simulink model "SIMULINK_FT_SRL_NZS_Tracking_R18b"  (R2018b)
settings: Solver=FixedStepAuto  StartTime=0.0  StopTime=sim_end_time  FixedStep=fixed_step_size  RelTol=1e-3
InitFcn:
  | start_uav_car_10
values from neighbouring files (symbols this model uses):
  a = 1    [start_uav_car_10.m]
  act_end = 2*pi/w1    (= 62.8318530718)    [start_uav_car_10.m]
  b = 1.8    [start_uav_car_10.m]
  battery_threshold = 20    [start_uav_car_10.m]
  bb = 1.2    [start_uav_car_10.m]
  delta_ = [delta_his(2:end,:); delta]    [adp_tracking.m]    (also in start_uav_car_10.m = zeros(N,1))
  draw_gif = false    [start_uav_car_10.m]
  fixed_step_size = 1/30    (= 0.0333333333333)    [start_uav_car_10.m]
  k = 0.2    [start_uav_car_10.m]
  KD_x = 0.000002    (= 2e-06)    [start_uav_car_10.m]
  KD_y = 0.00002    (= 2e-05)    [start_uav_car_10.m]
  kd_z = 0.02    [start_uav_car_10.m]
  KDD_x = 0.0008    [start_uav_car_10.m]
  KDD_y = 0.0008    [start_uav_car_10.m]
  KI_x = 0.000002    (= 2e-06)    [start_uav_car_10.m]
  KI_y = 0.000002    (= 2e-06)    [start_uav_car_10.m]
  ki_z = 0.002    [start_uav_car_10.m]
  KII_x = 0.000000    (= 0)    [start_uav_car_10.m]
  KII_y = 0.000    (= 0)    [start_uav_car_10.m]
  KP_x = 1.5    [start_uav_car_10.m]
  KP_y = 1.5    [start_uav_car_10.m]
  kp_z = 0.7    [start_uav_car_10.m]
  KPP_x = 0.4    [start_uav_car_10.m]
  KPP_y = 0.4    [start_uav_car_10.m]
  lmt = 0.5    [start_uav_car_10.m]
  omega = omega_(i,:)    [adp_tracking.m]    (also in start_uav_car_10.m = 0.3)
  omega_ = [omega_his(2:end,:); omega']    [adp_tracking.m]    (also in start_uav_car_10.m = zeros(N,l))
  R = 200*eye(2)    [adp_tracking.m]    (also in start_uav_car_10.m = 0.7)
  sim_end_time = 300    [start_uav_car_10.m]    (also in trjcar.m = 600)
  UAV_NUM = 1    [start_uav_car_10.m]
  Vel_Switch_1 = 1    [start_uav_car_10.m]
  Vel_Switch_10 = 1    [start_uav_car_10.m]
  Vel_Switch_11 = 1    [start_uav_car_10.m]
  Vel_Switch_12 = 1    [start_uav_car_10.m]
  Vel_Switch_13 = 1    [start_uav_car_10.m]
  Vel_Switch_14 = 1    [start_uav_car_10.m]
  Vel_Switch_15 = 1    [start_uav_car_10.m]
  Vel_Switch_16 = 1    [start_uav_car_10.m]
  Vel_Switch_17 = 1    [start_uav_car_10.m]
  Vel_Switch_18 = 1    [start_uav_car_10.m]
  Vel_Switch_19 = 1    [start_uav_car_10.m]
  Vel_Switch_2 = 1    [start_uav_car_10.m]
  Vel_Switch_20 = 1    [start_uav_car_10.m]
  Vel_Switch_3 = 1    [start_uav_car_10.m]
  Vel_Switch_4 = 1    [start_uav_car_10.m]
  Vel_Switch_5 = 1    [start_uav_car_10.m]
  Vel_Switch_6 = 1    [start_uav_car_10.m]
  Vel_Switch_7 = 1    [start_uav_car_10.m]
  Vel_Switch_8 = 1    [start_uav_car_10.m]
  Vel_Switch_9 = 1    [start_uav_car_10.m]
  W0 = 10*ones(l,1)    [start_uav_car_10.m]
  w1 = 0.1    [start_uav_car_10.m]
  w2 = 30    [start_uav_car_10.m]
  XMAX = 2.8    [start_uav_car_10.m]
  XMIN = -2.8    [start_uav_car_10.m]
  YMAX = 2.2    [start_uav_car_10.m]
  YMIN = -2.2    [start_uav_car_10.m]
  ys = ys_learned - ys_learned(1,:)    [start_uav_car_10.m]
  ys_learned = [-20 -19.9842645881 -19.9722755737 -19.9635643089 -19.9577075469 -19.9543235714 -19.9530686431 -19.9536337356 -19.9557415391 -19.9591437091 -19.9636183405 -19.9689676484 ... (12618 elements, 6309x2)]    [DMP_ref.mat]
  z_d_for_land = 1    [start_uav_car_10.m]
  ZMAX = 2.0    (= 2)    [start_uav_car_10.m]
  ZMIN = 0.7    [start_uav_car_10.m]
undefined symbols (not defined in the file or in its folder): droneyeeUAV2_NUM, droneyeeUAV3_NUM, droneyeeUAV4_NUM, droneyeeUAV5_NUM, uav10num, uav1num, uav2num, uav3num, uav4num, uav5num, uav6num, uav7num, uav8num, uav9num
libraries: simulink x121, aerolibanimutils x1
(part 11 of 11)

== matlab function SIMULINK_FT_SRL_NZS_Tracking_R18b/CMD_car1/CMD6/MATLAB Function1 ==
  settings: updateMethod=DISCRETE
  data: x_d input; y_d input; z_d input; timestamp input; x input; y input; z input; battery_status input; sim_time_end input; x_d_ output; battery_threshold input; z_d_for_land input; y_d_ output; z_d_ output; UAV_NUM input
function [x_d_, y_d_, z_d_] = fcn(x_d, y_d, z_d, timestamp, x,y,z,battery_status, sim_time_end,battery_threshold, z_d_for_land, UAV_NUM)
persistent s_x s_y s_z ready_land
if isempty(s_x)
    s_x = x;
end
if isempty(s_y)
    s_y = y;
end
if isempty(s_z)
    s_z = z;
end
if isempty(ready_land)
    ready_land = false;
end
    
battery_low = false;
for i = 1:UAV_NUM
    if battery_status(i) < battery_threshold
        battery_low = true;
        break;
    end
end
if sim_time_end - timestamp < 1
    tello_stop = true;
else
    tello_stop = false;
end
if battery_low || tello_stop
    if ~ready_land
        ready_land = true;
    end
    z_d_ = z_d_for_land;
    x_d_ = s_x;
    y_d_ = s_y;
else
   ready_land = false;
   s_x = x;
   s_y = y;
   x_d_ = x_d;
   y_d_ = y_d;
   z_d_ = z_d;
end

== matlab function SIMULINK_FT_SRL_NZS_Tracking_R18b/control system_UAV/MATLAB Function ==
  data: u input; y output
function y = fcn(u)
plot(u(1),u(2),"*");
hold on;
y = u;

== matlab function SIMULINK_FT_SRL_NZS_Tracking_R18b/防碰撞2/MATLAB Function ==
  settings: updateMethod=DISCRETE
  data: u1 input; xd output; u2 input; yd output; zd output; u3 input; u4 input; u5 input; flag input
function [xd,yd,zd] = fcn(u1,u2,u3,u4,u5,flag)
persistent xdd ydd zdd xtt ytt ztt;
k=u4;
totnum =10;
safedist =u3;%安全距离的平方
bang=u5;
xdd=zeros(totnum,1);
ydd=zeros(totnum,1);
zdd=zeros(totnum,1);
xt=zeros(totnum,1);
yt=zeros(totnum,1);
zt=zeros(totnum,1);
vx=xt;
vy=yt;
vz=zt;
xd=xt;
yd=yt;
zd=zt;
for i =1:1:totnum
    xt(i)=u2(12*(i-1)+1);
    yt(i)=u2(12*(i-1)+2);
    zt(i)=u2(12*(i-1)+3);
    xd(i)=u1(6*(i-1)+1);
    yd(i)=u1(6*(i-1)+2);
    zd(i)=u1(6*(i-1)+3);
    vx(i)=u2(12*(i-1)+10);
    vy(i)=u2(12*(i-1)+11);
    vz(i)=u2(12*(i-1)+12);
end
if flag==1
if isempty(xt)
    xtt = xt;
    ytt = yt;
    ztt = zt;
end
for i =1:1:(totnum-1)
    if xt(i)==0&&yt(i)==0&&zt(i)==0
        break
    end
    for j=(i+1):1:totnum
        if xt(j)==0&&yt(j)==0&&zt(j)==0
        break
        end
        dist=((xt(i)-xt(j))^2+(yt(i)-yt(j))^2+(zt(i)-zt(j))^2);
        sqrt_dist=sqrt((xt(i)-xt(j))^2+(yt(i)-yt(j))^2);
    if (dist>0)&&(sqrt(dist)<=bang)
%         xd(i)=xt(i);
%         yd(i)=yt(i);
%         zd(i)=0; %zt(i);
%         xd(j)=xt(j);
%         yd(j)=yt(j);
%         zd(j)=zt(j);        
%         xd(i)=xd(i)+k*(xt(i)-xt(j))*(safedist-dist);
%         yd(i)=yd(i)+k*(yt(i)-yt(j))*(safedist-dist);
        xdd(i)=xdd(i)+k*(xt(i)-xt(j))*(safedist-dist);
        ydd(i)=ydd(i)+k*(yt(i)-yt(j))*(safedist-dist);
%         zd(i)=zd(i)+k*(zt(i)-zt(j))*(safedist-dist);
%         xd(j)=xd(j)-k*(xt(i)-xt(j))*(safedist-dist);
%         yd(j)=yd(j)-k*(yt(i)-yt(j))*(safedist-dist);
        xdd(j)=xdd(j)-k*(xt(i)-xt(j))*(safedist-dist);
        ydd(j)=ydd(j)-k*(yt(i)-yt(j))*(safedist-dist);
%         zd(j)=zd(j)-k*(zt(i)-zt(j))*(safedist-dist);
     elseif (sqrt(dist)<safedist)&&(((vx(i)-vx(j))*(xt(i)-xt(j))+...
             (vy(i)-vy(j))*(yt(i)-yt(j)))<0)
%         dist=dist-bang;
%         xd(i)=xd(i)+k*(yt(i)-yt(j))*(safedist-dist);
%         yd(i)=yd(i)+k*(xt(j)-xt(i))*(safedist-dist);
        xdd(i)=xdd(i)+k*(yt(i)-yt(j))*(safedist-sqrt_dist)/sqrt_dist/sqrt_dist;
        ydd(i)=ydd(i)+k*(xt(j)-xt(i))*(safedist-sqrt_dist)/sqrt_dist/sqrt_dist;
%         zd(i)=zd(i)+k*(zt(i)-zt(j))*(safedist-dist);
%         xd(j)=xd(j)-k*(yt(i)-yt(j))*(safedist-dist);
%         yd(j)=yd(j)-k*(xt(j)-xt(i))*(safedist-dist);
        xdd(j)=xdd(j)-k*(yt(i)-yt(j))*(safedist-sqrt_dist)/sqrt_dist/sqrt_dist;
        ydd(j)=ydd(j)-k*(xt(j)-xt(i))*(safedist-sqrt_dist)/sqrt_dist/sqrt_dist;
%         zd(j)=zd(j)-k*(zt(i)-zt(j))*(safedist-dist);
        
    end
    end
end
xd=xd+xdd;
yd=yd+ydd;
% zd=zdd;
end

== matlab function SIMULINK_FT_SRL_NZS_Tracking_R18b/control system_UAV/Baseline Controller3/MATLAB Function ==
  data: u input; y output; a input
function y = fcn(u,a)
y = satgd(u,a);

== matlab function SIMULINK_FT_SRL_NZS_Tracking_R18b/CMD_car1/CMD6/Subsystem/MATLAB Function ==
  settings: updateMethod=DISCRETE
  data: timestamp input; uavnum input; x_ output; y_ output; z_ output; switch_flag input; stas input; trj_flag input; form_flag input; avo_flag input
function [x_, y_, z_] = fcn(timestamp, uavnum,switch_flag,stas,trj_flag,form_flag,avo_flag)

[x_,y_,z_]=trjcar(timestamp,uavnum,switch_flag,stas,trj_flag,form_flag,avo_flag);

== matlab function SIMULINK_FT_SRL_NZS_Tracking_R18b/control system_UAV/Baseline Controller4/MATLAB Function ==
  data: u input; y output; a input
function y = fcn(u,a)
y = satgd(u,a);

== matlab function SIMULINK_FT_SRL_NZS_Tracking_R18b/CMD_car1/CMD7/MATLAB Function1 ==
  settings: updateMethod=DISCRETE
  data: x_d input; y_d input; z_d input; timestamp input; x input; y input; z input; battery_status input; sim_time_end input; x_d_ output; battery_threshold input; z_d_for_land input; y_d_ output; z_d_ output; UAV_NUM input
function [x_d_, y_d_, z_d_] = fcn(x_d, y_d, z_d, timestamp, x,y,z,battery_status, sim_time_end,battery_threshold, z_d_for_land, UAV_NUM)
persistent s_x s_y s_z ready_land
if isempty(s_x)
    s_x = x;
end
if isempty(s_y)
    s_y = y;
end
if isempty(s_z)
    s_z = z;
end
if isempty(ready_land)
    ready_land = false;
end
    
battery_low = false;
for i = 1:UAV_NUM
    if battery_status(i) < battery_threshold
        battery_low = true;
        break;
    end
end
if sim_time_end - timestamp < 1
    tello_stop = true;
else
    tello_stop = false;
end
if battery_low || tello_stop
    if ~ready_land
        ready_land = true;
    end
    z_d_ = z_d_for_land;
    x_d_ = s_x;
    y_d_ = s_y;
else
   ready_land = false;
   s_x = x;
   s_y = y;
   x_d_ = x_d;
   y_d_ = y_d;
   z_d_ = z_d;
end

== matlab function SIMULINK_FT_SRL_NZS_Tracking_R18b/CMD_UAV/CMD6/Subsystem/MATLAB Function ==
  settings: updateMethod=DISCRETE
  data: timestamp input; uavnum input; x_ output; y_ output; z_ output; switch_flag input; stas input; trj_flag input; form_flag input; avo_flag input
function [x_, y_, z_] = fcn(timestamp, uavnum,switch_flag,stas,trj_flag,form_flag,avo_flag)

[x_,y_,z_]=trjuav(timestamp,uavnum,switch_flag,stas,trj_flag,form_flag,avo_flag);

== matlab function SIMULINK_FT_SRL_NZS_Tracking_R18b/CMD_UAV/CMD7/MATLAB Function1 ==
  settings: updateMethod=DISCRETE
  data: x_d input; y_d input; z_d input; timestamp input; x input; y input; z input; battery_status input; sim_time_end input; x_d_ output; battery_threshold input; z_d_for_land input; y_d_ output; z_d_ output; UAV_NUM input
function [x_d_, y_d_, z_d_] = fcn(x_d, y_d, z_d, timestamp, x,y,z,battery_status, sim_time_end,battery_threshold, z_d_for_land, UAV_NUM)
persistent s_x s_y s_z ready_land
if isempty(s_x)
    s_x = x;
end
if isempty(s_y)
    s_y = y;
end
if isempty(s_z)
    s_z = z;
end
if isempty(ready_land)
    ready_land = false;
end
    
battery_low = false;
for i = 1:UAV_NUM
    if battery_status(i) < battery_threshold
        battery_low = true;
        break;
    end
end
if sim_time_end - timestamp < 1
    tello_stop = true;
else
    tello_stop = false;
end
if battery_low || tello_stop
    if ~ready_land
        ready_land = true;
    end
    z_d_ = z_d_for_land;
    x_d_ = s_x;
    y_d_ = s_y;
else
   ready_land = false;
   s_x = x;
   s_y = y;
   x_d_ = x_d;
   y_d_ = y_d;
   z_d_ = z_d;
end

== matlab function SIMULINK_FT_SRL_NZS_Tracking_R18b/CMD_UAV/CMD7/Subsystem/MATLAB Function ==
  settings: updateMethod=DISCRETE
  data: timestamp input; uavnum input; x_ output; y_ output; z_ output; switch_flag input; stas input; trj_flag input; form_flag input; avo_flag input
function [x_, y_, z_] = fcn(timestamp, uavnum,switch_flag,stas,trj_flag,form_flag,avo_flag)

[x_,y_,z_]=trjuav(timestamp,uavnum,switch_flag,stas,trj_flag,form_flag,avo_flag);

== matlab function SIMULINK_FT_SRL_NZS_Tracking_R18b/CMD_UAV/CMD8/MATLAB Function1 ==
  settings: updateMethod=DISCRETE
  data: x_d input; y_d input; z_d input; timestamp input; x input; y input; z input; battery_status input; sim_time_end input; x_d_ output; battery_threshold input; z_d_for_land input; y_d_ output; z_d_ output; UAV_NUM input
function [x_d_, y_d_, z_d_] = fcn(x_d, y_d, z_d, timestamp, x,y,z,battery_status, sim_time_end,battery_threshold, z_d_for_land, UAV_NUM)
persistent s_x s_y s_z ready_land
if isempty(s_x)
    s_x = x;
end
if isempty(s_y)
    s_y = y;
end
if isempty(s_z)
    s_z = z;
end
if isempty(ready_land)
    ready_land = false;
end
    
battery_low = false;
for i = 1:UAV_NUM
    if battery_status(i) < battery_threshold
        battery_low = true;
        break;
    end
end
if sim_time_end - timestamp < 1
    tello_stop = true;
else
    tello_stop = false;
end
if battery_low || tello_stop
    if ~ready_land
        ready_land = true;
    end
    z_d_ = z_d_for_land;
    x_d_ = s_x;
    y_d_ = s_y;
else
   ready_land = false;
   s_x = x;
   s_y = y;
   x_d_ = x_d;
   y_d_ = y_d;
   z_d_ = z_d;
end

== matlab function SIMULINK_FT_SRL_NZS_Tracking_R18b/CMD_UAV/CMD8/Subsystem/MATLAB Function ==
  settings: updateMethod=DISCRETE
  data: timestamp input; uavnum input; x_ output; y_ output; z_ output; switch_flag input; stas input; trj_flag input; form_flag input; avo_flag input
function [x_, y_, z_] = fcn(timestamp, uavnum,switch_flag,stas,trj_flag,form_flag,avo_flag)

[x_,y_,z_]=trjuav(timestamp,uavnum,switch_flag,stas,trj_flag,form_flag,avo_flag);

== matlab function SIMULINK_FT_SRL_NZS_Tracking_R18b/CMD_UAV/CMD10/MATLAB Function1 ==
  settings: updateMethod=DISCRETE
  data: x_d input; y_d input; z_d input; timestamp input; x input; y input; z input; battery_status input; sim_time_end input; x_d_ output; battery_threshold input; z_d_for_land input; y_d_ output; z_d_ output; UAV_NUM input
function [x_d_, y_d_, z_d_] = fcn(x_d, y_d, z_d, timestamp, x,y,z,battery_status, sim_time_end,battery_threshold, z_d_for_land, UAV_NUM)
persistent s_x s_y s_z ready_land
if isempty(s_x)
    s_x = x;
end
if isempty(s_y)
    s_y = y;
end
if isempty(s_z)
    s_z = z;
end
if isempty(ready_land)
    ready_land = false;
end
    
battery_low = false;
for i = 1:UAV_NUM
    if battery_status(i) < battery_threshold
        battery_low = true;
        break;
    end
end
if sim_time_end - timestamp < 1
    tello_stop = true;
else
    tello_stop = false;
end
if battery_low || tello_stop
    if ~ready_land
        ready_land = true;
    end
    z_d_ = z_d_for_land;
    x_d_ = s_x;
    y_d_ = s_y;
else
   ready_land = false;
   s_x = x;
   s_y = y;
   x_d_ = x_d;
   y_d_ = y_d;
   z_d_ = z_d;
end

== matlab function SIMULINK_FT_SRL_NZS_Tracking_R18b/CMD_UAV/CMD10/Subsystem/MATLAB Function ==
  settings: updateMethod=DISCRETE
  data: timestamp input; uavnum input; x_ output; y_ output; z_ output; switch_flag input; stas input; trj_flag input; form_flag input; avo_flag input
function [x_, y_, z_] = fcn(timestamp, uavnum,switch_flag,stas,trj_flag,form_flag,avo_flag)

[x_,y_,z_]=trjuav(timestamp,uavnum,switch_flag,stas,trj_flag,form_flag,avo_flag);

== matlab function SIMULINK_FT_SRL_NZS_Tracking_R18b/CMD_UAV/CMD9/MATLAB Function1 ==
  settings: updateMethod=DISCRETE
  data: x_d input; y_d input; z_d input; timestamp input; x input; y input; z input; battery_status input; sim_time_end input; x_d_ output; battery_threshold input; z_d_for_land input; y_d_ output; z_d_ output; UAV_NUM input
function [x_d_, y_d_, z_d_] = fcn(x_d, y_d, z_d, timestamp, x,y,z,battery_status, sim_time_end,battery_threshold, z_d_for_land, UAV_NUM)
persistent s_x s_y s_z ready_land
if isempty(s_x)
    s_x = x;
end
if isempty(s_y)
    s_y = y;
end
if isempty(s_z)
    s_z = z;
end
if isempty(ready_land)
    ready_land = false;
end
    
battery_low = false;
for i = 1:UAV_NUM
    if battery_status(i) < battery_threshold
        battery_low = true;
        break;
    end
end
if sim_time_end - timestamp < 1
    tello_stop = true;
else
    tello_stop = false;
end
if battery_low || tello_stop
    if ~ready_land
        ready_land = true;
    end
    z_d_ = z_d_for_land;
    x_d_ = s_x;
    y_d_ = s_y;
else
   ready_land = false;
   s_x = x;
   s_y = y;
   x_d_ = x_d;
   y_d_ = y_d;
   z_d_ = z_d;
end

== matlab function SIMULINK_FT_SRL_NZS_Tracking_R18b/CMD_UAV/CMD9/Subsystem/MATLAB Function ==
  settings: updateMethod=DISCRETE
  data: timestamp input; uavnum input; x_ output; y_ output; z_ output; switch_flag input; stas input; trj_flag input; form_flag input; avo_flag input
function [x_, y_, z_] = fcn(timestamp, uavnum,switch_flag,stas,trj_flag,form_flag,avo_flag)

[x_,y_,z_]=trjuav(timestamp,uavnum,switch_flag,stas,trj_flag,form_flag,avo_flag);

== matlab function SIMULINK_FT_SRL_NZS_Tracking_R18b/CMD_car1/CMD7/Subsystem/MATLAB Function ==
  settings: updateMethod=DISCRETE
  data: timestamp input; uavnum input; x_ output; y_ output; z_ output; switch_flag input; stas input; trj_flag input; form_flag input; avo_flag input
function [x_, y_, z_] = fcn(timestamp, uavnum,switch_flag,stas,trj_flag,form_flag,avo_flag)

[x_,y_,z_]=trjcar(timestamp,uavnum,switch_flag,stas,trj_flag,form_flag,avo_flag);

== matlab function SIMULINK_FT_SRL_NZS_Tracking_R18b/CMD_car1/CMD8/MATLAB Function1 ==
  settings: updateMethod=DISCRETE
  data: x_d input; y_d input; z_d input; timestamp input; x input; y input; z input; battery_status input; sim_time_end input; x_d_ output; battery_threshold input; z_d_for_land input; y_d_ output; z_d_ output; UAV_NUM input
function [x_d_, y_d_, z_d_] = fcn(x_d, y_d, z_d, timestamp, x,y,z,battery_status, sim_time_end,battery_threshold, z_d_for_land, UAV_NUM)
persistent s_x s_y s_z ready_land
if isempty(s_x)
    s_x = x;
end
if isempty(s_y)
    s_y = y;
end
if isempty(s_z)
    s_z = z;
end
if isempty(ready_land)
    ready_land = false;
end
    
battery_low = false;
for i = 1:UAV_NUM
    if battery_status(i) < battery_threshold
        battery_low = true;
        break;
    end
end
if sim_time_end - timestamp < 1
    tello_stop = true;
else
    tello_stop = false;
end
if battery_low || tello_stop
    if ~ready_land
        ready_land = true;
    end
    z_d_ = z_d_for_land;
    x_d_ = s_x;
    y_d_ = s_y;
else
   ready_land = false;
   s_x = x;
   s_y = y;
   x_d_ = x_d;
   y_d_ = y_d;
   z_d_ = z_d;
end

== matlab function SIMULINK_FT_SRL_NZS_Tracking_R18b/CMD_car1/CMD8/Subsystem/MATLAB Function ==
  settings: updateMethod=DISCRETE
  data: timestamp input; uavnum input; x_ output; y_ output; z_ output; switch_flag input; stas input; trj_flag input; form_flag input; avo_flag input
function [x_, y_, z_] = fcn(timestamp, uavnum,switch_flag,stas,trj_flag,form_flag,avo_flag)

[x_,y_,z_]=trjcar(timestamp,uavnum,switch_flag,stas,trj_flag,form_flag,avo_flag);

== matlab function SIMULINK_FT_SRL_NZS_Tracking_R18b/CMD_car1/CMD9/MATLAB Function1 ==
  settings: updateMethod=DISCRETE
  data: x_d input; y_d input; z_d input; timestamp input; x input; y input; z input; battery_status input; sim_time_end input; x_d_ output; battery_threshold input; z_d_for_land input; y_d_ output; z_d_ output; UAV_NUM input
function [x_d_, y_d_, z_d_] = fcn(x_d, y_d, z_d, timestamp, x,y,z,battery_status, sim_time_end,battery_threshold, z_d_for_land, UAV_NUM)
persistent s_x s_y s_z ready_land
if isempty(s_x)
    s_x = x;
end
if isempty(s_y)
    s_y = y;
end
if isempty(s_z)
    s_z = z;
end
if isempty(ready_land)
    ready_land = false;
end
    
battery_low = false;
for i = 1:UAV_NUM
    if battery_status(i) < battery_threshold
        battery_low = true;
        break;
    end
end
if sim_time_end - timestamp < 1
    tello_stop = true;
else
    tello_stop = false;
end
if battery_low || tello_stop
    if ~ready_land
        ready_land = true;
    end
    z_d_ = z_d_for_land;
    x_d_ = s_x;
    y_d_ = s_y;
else
   ready_land = false;
   s_x = x;
   s_y = y;
   x_d_ = x_d;
   y_d_ = y_d;
   z_d_ = z_d;
end

== matlab function SIMULINK_FT_SRL_NZS_Tracking_R18b/CMD_car1/CMD9/Subsystem/MATLAB Function ==
  settings: updateMethod=DISCRETE
  data: timestamp input; uavnum input; x_ output; y_ output; z_ output; switch_flag input; stas input; trj_flag input; form_flag input; avo_flag input
function [x_, y_, z_] = fcn(timestamp, uavnum,switch_flag,stas,trj_flag,form_flag,avo_flag)

[x_,y_,z_]=trjcar(timestamp,uavnum,switch_flag,stas,trj_flag,form_flag,avo_flag);

== matlab function SIMULINK_FT_SRL_NZS_Tracking_R18b/control system_car1/Baseline Controller1/MATLAB Function ==
  data: u input; y output; a input
function y = fcn(u,a)
y = satgd(u,a);

== matlab function SIMULINK_FT_SRL_NZS_Tracking_R18b/control system_car1/Baseline Controller2/MATLAB Function ==
  data: u input; y output; a input
function y = fcn(u,a)
y = satgd(u,a);

== matlab function SIMULINK_FT_SRL_NZS_Tracking_R18b/control system_car1/Baseline Controller3/MATLAB Function ==
  data: u input; y output; a input
function y = fcn(u,a)
y = satgd(u,a);

== matlab function SIMULINK_FT_SRL_NZS_Tracking_R18b/control system_car1/Baseline Controller4/MATLAB Function ==
  data: u input; y output; a input
function y = fcn(u,a)
y = satgd(u,a);

== matlab function SIMULINK_FT_SRL_NZS_Tracking_R18b/control system_car1/Baseline Controller5/MATLAB Function ==
  data: u input; y output; a input
function y = fcn(u,a)
y = satgd(u,a);

== matlab function SIMULINK_FT_SRL_NZS_Tracking_R18b/control system_car1/MATLAB Function ==
  data: u input; y output
function y = fcn(u)
plot(u(1),u(2),"*");
hold on;
y = u;

== matlab function SIMULINK_FT_SRL_NZS_Tracking_R18b/control system_car1/Baseline Controller6/MATLAB Function ==
  data: u input; y output; a input
function y = fcn(u,a)
y = satgd(u,a);

== matlab function SIMULINK_FT_SRL_NZS_Tracking_R18b/control system_car1/Baseline Controller7/MATLAB Function ==
  data: u input; y output; a input
function y = fcn(u,a)
y = satgd(u,a);

== matlab function SIMULINK_FT_SRL_NZS_Tracking_R18b/control system_car1/Baseline Controller8/MATLAB Function ==
  data: u input; y output; a input
function y = fcn(u,a)
y = satgd(u,a);

== matlab function SIMULINK_FT_SRL_NZS_Tracking_R18b/control system_car1/Baseline Controller9/MATLAB Function ==
  data: u input; y output; a input
function y = fcn(u,a)
y = satgd(u,a);

== matlab function SIMULINK_FT_SRL_NZS_Tracking_R18b/防碰撞1/MATLAB Function1 ==
  settings: updateMethod=DISCRETE
  data: u1 input; xd output; u2 input; yd output; zd output; u3 input; u4 input; u5 input; flag input
function [xd,yd,zd] = fcn(u1,u2,u3,u4,u5,flag)

persistent xdd ydd zdd xtt ytt ztt;
k=u4;
totnum =10;
safedist =u3;%安全距离
bang=u5;
xdd=zeros(totnum,1);
ydd=zeros(totnum,1);
zdd=zeros(totnum,1);
xt=zeros(totnum,1);
yt=zeros(totnum,1);
zt=zeros(totnum,1);
vx=xt;
vy=yt;
vz=zt;
xd=xt;
yd=yt;
zd=zt;

for i =1:1:totnum
    xt(i)=u2(12*(i-1)+1);
    yt(i)=u2(12*(i-1)+2);
    zt(i)=u2(12*(i-1)+3);
    vx(i)=u2(12*(i-1)+10);
    vy(i)=u2(12*(i-1)+11);
    vz(i)=u2(12*(i-1)+12);
    xd(i)=u1(4*(i-1)+1);
    yd(i)=u1(4*(i-1)+2);
    zd(i)=u1(4*(i-1)+3);
end
if flag==1
    if isempty(xtt)
        xtt = xt;
        ytt = yt;
        ztt = zt;
    end
    for i =1:1:(totnum-1)
        if (xt(i)==0)&&(yt(i)==0)&&(zt(i)==0)
            continue
        end
        for j=(i+1):1:totnum
            if xt(j)==0 && yt(j)==0 && zt(j)==0
                continue
            end
            dist=(xt(i)-xt(j))^2+(yt(i)-yt(j))^2+(zt(i)-zt(j))^2;
            sqrt_dist=sqrt((xt(i)-xt(j))^2+(yt(i)-yt(j))^2);
            if (dist>0)&&(sqrt(dist)<bang)
                %         xdd(i)=xtt(i);
                %         ydd(i)=ytt(i);
                %         zdd(i)=ztt(i);
                %         xdd(j)=xtt(j);
                %         ydd(j)=ytt(j);
                %         zdd(j)=ztt(j);
                xdd(i)=k*(xt(i)-xt(j))*(safedist-sqrt_dist)/dist;
                ydd(i)=k*(yt(i)-yt(j))*(safedist-sqrt_dist)/dist;
                %         zdd(i)=zt(i)+k*(zt(i)-zt(j))*(safedist-sqrt_dist)/sqrt_dist;
                xdd(j)=-k*(xt(i)-xt(j))*(safedist-sqrt_dist)/dist;
                ydd(j)=-k*(yt(i)-yt(j))*(safedist-sqrt_dist)/dist;
                %         zdd(j)=zt(j)-k*(zt(i)-zt(j))*(safedist-dist)/sqrt_dist;
                
            elseif (sqrt(dist)<safedist)&&(((vx(i)-vx(j))*(xt(i)-xt(j))+...
                    (vy(i)-vy(j))*(yt(i)-yt(j)))<0)
                %         xdd(i)=(xdd(i)+xt(i)+k*(yt(i)-yt(j))*(safedist-sqrt_dist)/dist)/(k*(safedist-sqrt_dist)/dist+1);
                %         ydd(i)=(ydd(i)+yt(i)+k*(xt(j)-xt(i))*(safedist-sqrt_dist)/dist)/(k*(safedist-sqrt_dist)/dist+1);
                %         zdd(i)=zdd(i)+k*(zt(i)-zt(j))*(safedist-sqrt_dist)/sqrt_dist;
                %         xdd(j)=(xdd(j)+xt(j)-k*(yt(i)-yt(j))*(safedist-sqrt_dist)/dist)/(k*(safedist-sqrt_dist)/dist+1);
                %         ydd(j)=(ydd(j)+yt(j)-k*(xt(j)-xt(i))*(safedist-sqrt_dist)/dist)/(k*(safedist-sqrt_dist)/dist+1);
                %         zdd(j)=zdd(j)-k*(zt(i)-zt(j))*(safedist-sqrt_dist)/sqrt_dist;
                %
                %         xdd(i)=(xt(i)+k*(yt(i)-yt(j))*(safedist-sqrt_dist)/dist)/(k*(safedist-sqrt_dist)/dist+1);
                %         ydd(i)=(yt(i)+k*(xt(j)-xt(i))*(safedist-sqrt_dist)/dist)/(k*(safedist-sqrt_dist)/dist+1);
                %         zdd(i)=zdd(i)+k*(zt(i)-zt(j))*(safedist-sqrt_dist)/sqrt_dist;
                %         xdd(j)=(xt(j)-k*(yt(i)-yt(j))*(safedist-sqrt_dist)/dist)/(k*(safedist-sqrt_dist)/dist+1);
                %         ydd(j)=(yt(j)-k*(xt(j)-xt(i))*(safedist-sqrt_dist)/dist)/(k*(safedist-sqrt_dist)/dist+1);
                %         zdd(j)=zdd(j)-k*(zt(i)-zt(j))*(safedist-sqrt_dist)/sqrt_dist;
                
                xdd(i)=(xdd(i)+k*(yt(i)-yt(j))*(safedist-sqrt_dist)/dist);
                ydd(i)=(ydd(i)+k*(xt(j)-xt(i))*(safedist-sqrt_dist)/dist);
                %         zdd(i)=zdd(i)+k*(zt(i)-zt(j))*(safedist-sqrt_dist)/sqrt_dist;
                xdd(j)=(xdd(j)-k*(yt(i)-yt(j))*(safedist-sqrt_dist)/dist);
                ydd(j)=(ydd(j)-k*(xt(j)-xt(i))*(safedist-sqrt_dist)/dist);
                %         zdd(j)=zdd(j)-k*(zt(i)-zt(j))*(safedist-sqrt_dist)/sqrt_dist;
                
            end
        end
        
    end
    
    for m =1:1:totnum
        if (xdd(m) ~= 0)||(ydd(m)~= 0)
            xd(m)=xdd(m)+xt(m);
            yd(m)=ydd(m)+yt(m);
        end
    end
    % zd=zdd;
    
    
end
end

== matlab function SIMULINK_FT_SRL_NZS_Tracking_R18b/control system_car1/Baseline Controller10/MATLAB Function ==
  data: u input; y output; a input
function y = fcn(u,a)
y = satgd(u,a);

== matlab function SIMULINK_FT_SRL_NZS_Tracking_R18b/control system_UAV/Baseline Controller3/Position controller/MATLAB Function ==
  data: x input; p output; y input
function p = fcn(x,y)

p = [x;y];

== matlab function SIMULINK_FT_SRL_NZS_Tracking_R18b/control system_UAV/Baseline Controller3/Position controller/MATLAB Function1 ==
  data: x input; p output; y input
function p = fcn(x,y)

p = [x;y];

== matlab function SIMULINK_FT_SRL_NZS_Tracking_R18b/control system_UAV/Baseline Controller3/Position controller/X-Y ADP tracking controller/DMP_ref ==
  data: t input; u input; y output
function y = fcn(t,u)
N = length(u);
if t < 12
    y = [0,0]';
elseif t < 12+N*0.01 -1
    i = floor((t-12)/0.01)+1;
    y = (u(i,:)-u(1,:))';
else
    y = (u(end,:)-u(1,:))';
end
% y = y';

== matlab function SIMULINK_FT_SRL_NZS_Tracking_R18b/control system_UAV/Baseline Controller3/Position controller/X-Y ADP tracking controller/Obstacle detection ==
  data: X input; y output; Cache1 output
function [y,Cache1] = LCOA(X)
P_wp1=[10;30];  % target location

% x = X(1:2)-P_wp1;
x = X(1:2);
ro = 0.3;
ra = ro * 2;
rd = ro * 3;
L1 = 0.3; L2 = 0.8; L3 = 0.2;

% zk_ = [10 18; 18 18]-[P_wp1';P_wp1'];
% zk_ = [9-0.5 15; 17-0.5 15];
% zk_ = [9-1 15; 17-1 15];
% zk_ = [9-2 15; 17-2 15];
% zk_ = [1 15; 9 15];
% zk_ = [1.5 15; 8.5 15];
% zk_ = [2 15; 8 15];
% zk_ = [3 12; 7 18];
% zk_ = [3+0.5 15; 9 15];
% zk_ = [9 10; 11.5 25];
% zk_ = [10.5 15; 11.5 25];
% zk_ = [-1.8 -0.6; -0.8 0.5];

% 241124
% zk_ = [-1.2 0; 8 0.5];
% zk_ = [-4 0; 8 0.5];
zk_ = [-1.2 0; 8 0.5];

s = 0; ds = [0;0];
beta = 0; dbeta = [0;0];

for i = 1:length(zk_)
    zk = zk_(i,:)';
    dk = norm(x-zk);
    ddk = (x-zk)/dk;
    betak = dk - ro;
    dbetak = ddk;
    
    if dk > rd
        sk = 0;
        dsk = [0;0];
    elseif dk >ra
        sk = L1 + L1 * cos(pi*(dk^2 - ra^2)/(rd^2 - ra^2));
        dsk = -2*pi*dk*ddk*sin(pi*(dk^2 - ra^2)/(rd^2 - ra^2))/(rd^2 - ra^2);
    elseif dk > ro
        sk = L2 + L3 * cos(pi*(dk^2 - ro^2)/(ra^2 - ro^2));
        dsk = -2*pi*dk*ddk*sin(pi*(dk^2 - ro^2)/(ra^2 - ro^2))/(ra^2 - ro^2);
    else
        sk = 1;
        dsk = [0;0];
    end
    ds = ds + dsk; s = s + sk;
    dbeta = dbeta + dbetak;
    beta = beta + betak;
end

mu = 0.01;
Kb = 20;
% Kb = 20;
% y = Kb * (dsk *(betak + mu) - dbetak * sk)/(betak + mu)^2; 
y = Kb * (ds *(beta + mu) - dbeta * s)/(beta + mu)^2; 


P_wp1=[10;30];  % target location

rrr=[ro;ra;rd];
Cache1=[rrr;P_wp1;zk_(1,:)';zk_(2,:)']; % input for plot111.m

== matlab function SIMULINK_FT_SRL_NZS_Tracking_R18b/control system_UAV/Baseline Controller3/Position controller/X-Y ADP tracking controller/adp_tracking ==
  data: P_feedback1 input; ux1 output; p_virtual1 input; Joystick input; delta_his input; omega_his input; delta2_his input; W input; W2 input; t input; dP_feedback1 input; lcoa input; uy1 output; ux2 output; uy2 output; delta_ output; omega_ output; delta2_ output; dW_ output; dW2_ output; test output
function [ux1,uy1,ux2,uy2,delta_, omega_, delta2_,dW_,dW2_,test] = adp_tracking(P_feedback1,p_virtual1,Joystick,delta_his,omega_his,delta2_his,W,W2,t,dP_feedback1,lcoa)
% the parameter of 'approaching'

% P_wp1=[10;30];  % target location

sampleTime = 1/25;
g = 9.8;
A = zeros(2);
B = eye(2)/g;
% B = [zeros(2);eye(2)]/g;
Q = 100*eye(2);
% R = 50*eye(2);
R = 25*eye(2);
R2 = R*2;
Q2 = Q/2;
l = length(W);

dx = dP_feedback1;
% dx = u;

%% ADP Path Planning

% x = P_feedback1 - P_wp1;
x = P_feedback1 - p_virtual1;
x1 = x(1); x2 = x(2);
% phi = [x1^2;x1*x2;x2^2];
% dphi = [2*x1 0; x2 x1; 0 2*x2];
% [sig,sig_p] = Staf_Basis(x); % State-following NN basis
alpha = 0.8;
% alpha = 1;
sig_p = Grad_Sigma_V_FT(x,alpha);
dphi = sig_p;
test = norm(dphi);


%% update
% W = 1*[30.7119   42.8391  115.4889]';
umax = 1;
u_adp = -umax*tanh(0.5/umax*R\B'*dphi'*W);
u2_adp = -umax*tanh(0.5/umax*R2\B'*dphi'*W2);
% u_adp = -0.5*R\B'*dphi'*W;
u_safe = -0.5*R\B*lcoa;
u2_safe = -0.5*R2\B*lcoa;
u_adp = u_adp + u_safe;% + u_human;
u2_adp = u2_adp + u2_safe;% + u_human;
% u_adp = -0.5*R\B'*dphi'*W;
% u_adp = lambda * u_adp + (1-lambda) * u_safe;
% K_lqr = [0.7071 0.0000; 0.0000 0.7071]*2;
% u_adp = -K_lqr*x;

if t > 10
%     u = u_adp;
%     u = -0.5*R\B'*dphi'*W;
    u = -umax*tanh(0.5/umax*R\B'*dphi'*W);
    u2 = -umax*tanh(0.5/umax*R2\B'*dphi'*W2);
else
    u = zeros(2,1);
    u2 = zeros(2,1);
end
%% ADP nn

omega = dphi*dx;
rou = 1 + omega'*omega;

delta = W'*omega + x'*Q*x + u'*R*u + u2'*R*u2;
delta_ = [delta_his(2:end,:); delta];

delta2 = W2'*omega + x'*Q2*x + u2'*R2*u2 + u'*R2*u;
delta2_ = [delta2_his(2:end,:); delta2];

omega_ = [omega_his(2:end,:); omega'];


%% Concurrent learning
con_flag = 0;
if con_flag == 1 && t>10
    temp = zeros(l,1);
    for i = 1:length(delta_his)
        omega = omega_(i,:);
        delta = delta_(i,:);
        rou = 1 + omega*omega';
        temp = temp - 0.01*omega'./rou^2*delta; 
    end
    dW_ = temp;
elseif t>10
        dW_ = - 1*omega*delta/rou; 
        dW2_ = - 1*omega*delta2/rou; 
else
        dW_ = zeros(l,1);
        dW2_ = zeros(l,1);
end
%% 输出
% u_adp = u;
ux1 = u_adp(1);
uy1 = u_adp(2);

ux2 = u2_adp(1);
uy2 = u2_adp(2);

== matlab function SIMULINK_FT_SRL_NZS_Tracking_R18b/control system_UAV/Baseline Controller3/Position controller/X-Y ADP tracking controller/reference_traj ==
  data: t input; p_ref input; dp_ref output; u_adp output
function [dp_ref,u_adp] = reference_traj(t,p_ref)
g = 9.8;
A = zeros(2);
B = eye(2)/g;
Q = 10*eye(2);
% R = 10*eye(2);
R = 100*eye(2);

P_wp1=[10;30];  % target location
x = p_ref - P_wp1;
x1 = x(1); x2 = x(2);

phi = [x1^2;x1*x2;x2^2];
dphi = [2*x1 0; x2 x1; 0 2*x2];
% [sig,sig_p] = Staf_Basis(x); % State-following NN basis
% dphi = sig_p;
umax = 15;

% W = [69.6962  194.1919  732.3164]';
% W = [240.3627  511.9875  480.4859]';
% W = [626.9039  661.0018  523.60190]';
W = [161.9089  606.9426  710.8552]';
% u_adp = -0.5*R\B'*dphi'*W;
if t > 12
    u_adp = -umax*tanh(0.5/umax*R\B'*dphi'*W);
else
    u_adp = zeros(2,1);
end
dp_ref = A*p_ref + B*u_adp;
